simulink subsystem "PieroControladoSz"  (R2023b)
settings: Solver=VariableStepAuto  StartTime=0.0  StopTime=10.0  RelTol=1e-3
settings Model: Creator=adria  LastModifiedBy=adria

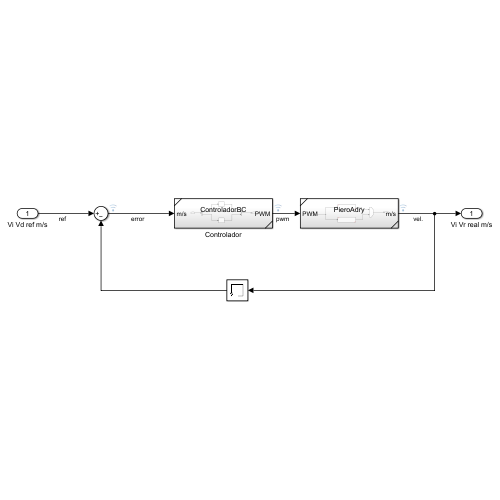
[thumbnail: Simulink's stored preview of the top-level diagram]
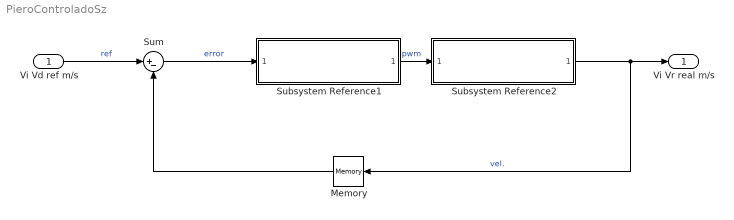
== system PieroControladoSz ==
  Vi Vd ref m/s : Inport  OutDataTypeStr=double  PortDimensions=2
  Memory : Memory
  Subsystem Reference1 : Subsystem  ReferencedSubsystem=ControladorBCz
  Subsystem Reference2 : Subsystem  ReferencedSubsystem=PieroAdryZ
  Sum : Sum  Inputs=|+-
  Vi Vr real m/s : Outport  OutDataTypeStr=double  PortDimensions=2
  wires:
  Sum/1 -> Subsystem Reference1/1  "error"
  Subsystem Reference2/1 -> Vi Vr real m/s/1, Memory/1  "vel."
  Subsystem Reference1/1 -> Subsystem Reference2/1  "pwm"
  Vi Vd ref m/s/1 -> Sum/1  "ref"
  Memory/1 -> Sum/2
